simulink model "linkageTest"  (R2020b)
settings: Solver=VariableStepAuto  StartTime=0.0  StopTime=90  RelTol=1e-3
libraries: simulink x1
settings Model: Creator=Edward  LastModifiedBy=Edward

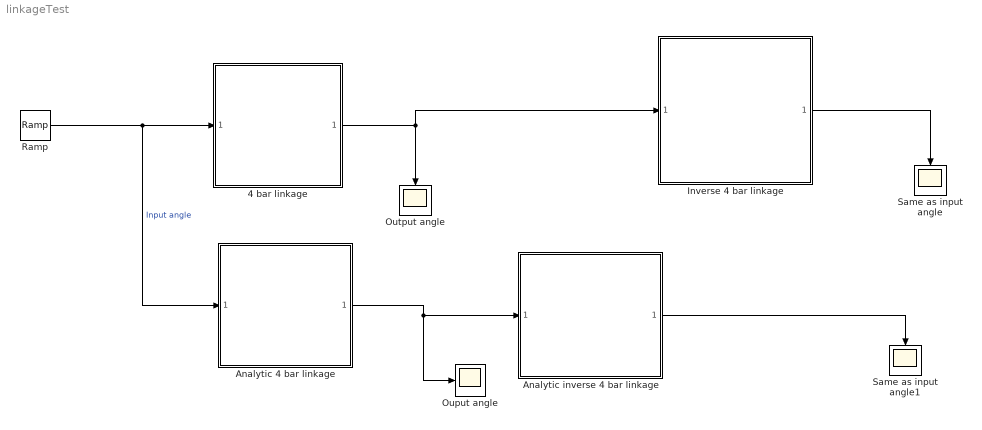
== system linkageTest ==
  4 bar linkage : Subsystem  ReferencedSubsystem=FourBarLinkage  g=21  a=10.17  h=30.625  b=20.78
  Analytic 4 bar linkage : Subsystem  ReferencedSubsystem=AnalyticFourBarLinkage  g=21  a=10.17  h=30.625  b=20.78  solutionSelector=1
  Analytic inverse 4 bar linkage : Subsystem  ReferencedSubsystem=AnalyticInverseFourBarLinkage  g=21  a=10.17  h=30.625  b=20.78  solutionSelector=1
  Inverse 4 bar linkage : Subsystem  ReferencedSubsystem=FlippedFourBarLinkage  g=21  a=10.17  h=30.625  b=20.78
  Ouput angle : Scope
  Output angle : Scope
  Ramp : simulink/Sources/Ramp  slope=2  start=0  InitialOutput=19
  Same as input angle : Scope
  Same as input angle1 : Scope
  wires:
  Ramp/1 -> Analytic 4 bar linkage/1, 4 bar linkage/1  "Input angle"
  4 bar linkage/1 -> Inverse 4 bar linkage/1, Output angle/1
  Inverse 4 bar linkage/1 -> Same as input angle/1
  Analytic 4 bar linkage/1 -> Analytic inverse 4 bar linkage/1, Ouput angle/1
  Analytic inverse 4 bar linkage/1 -> Same as input angle1/1
